simulink model "Switching_07"  (R2022b)
settings: Solver=ode4  StartTime=0.0  StopTime=50  FixedStep=1e-3  MaxStep=1e-3  RelTol=1e-3
undefined symbols (not defined in the file or in its folder): den_filter, der_sat, num_filter, OF_k1_FD, OF_k2_FD, OF_k3_FD, OF_k4_FD, p1, p2, p3, PR_k1, PR_k2, PR_k3, theta_d, tolerance_posture, v_sat, w_sat, x_d, y_d
libraries: simulink x18, dspsigops x3
settings Model: Creator=david  LastModifiedBy=aless

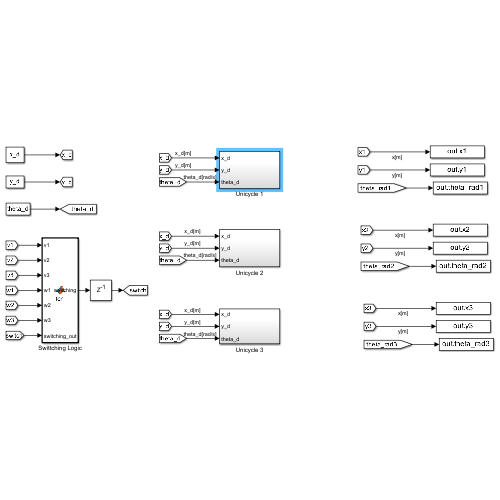
[thumbnail: Simulink's stored preview of the top-level diagram]
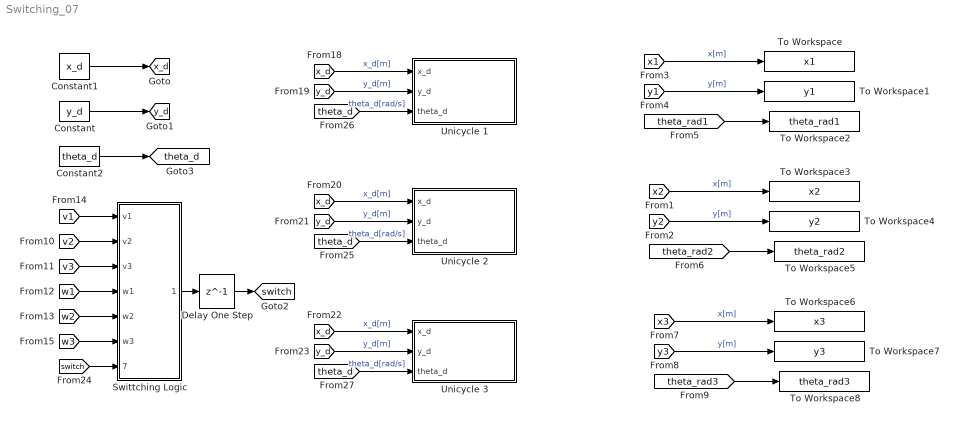
== system Switching_07 ==
  Constant : Constant  Value=y_d
  Constant1 : Constant  Value=x_d
  Constant2 : Constant  Value=theta_d
  Delay One Step : Delay  DelayLength=1
  Swittching Logic : MATLAB Function  TreatAsAtomicUnit=on
  To Workspace : ToWorkspace  VariableName=x1  SaveFormat=Structure With Time  SampleTime=-1
  To Workspace1 : ToWorkspace  VariableName=y1  SaveFormat=Structure With Time  SampleTime=-1
  To Workspace2 : ToWorkspace  VariableName=theta_rad1  SaveFormat=Structure With Time  SampleTime=-1
  To Workspace3 : ToWorkspace  VariableName=x2  SaveFormat=Structure With Time  SampleTime=-1
  To Workspace4 : ToWorkspace  VariableName=y2  SaveFormat=Structure With Time  SampleTime=-1
  To Workspace5 : ToWorkspace  VariableName=theta_rad2  SaveFormat=Structure With Time  SampleTime=-1
  To Workspace6 : ToWorkspace  VariableName=x3  SaveFormat=Structure With Time  SampleTime=-1
  To Workspace7 : ToWorkspace  VariableName=y3  SaveFormat=Structure With Time  SampleTime=-1
  To Workspace8 : ToWorkspace  VariableName=theta_rad3  SaveFormat=Structure With Time  SampleTime=-1
  Unicycle 1 : Subsystem
  Unicycle 2 : Subsystem
  Unicycle 3 : Subsystem
  tag scope: switch=global, theta_d=global, x_d=global, y_d=global
  wires:
  [x1] -> To Workspace/1  "x[m]"
  [y1] -> To Workspace1/1  "y[m]"
  [theta_rad1] -> To Workspace2/1
  [x2] -> To Workspace3/1  "x[m]"
  [y2] -> To Workspace4/1  "y[m]"
  [theta_rad2] -> To Workspace5/1
  [theta_rad3] -> To Workspace8/1
  [y3] -> To Workspace7/1  "y[m]"
  [x3] -> To Workspace6/1  "x[m]"
  [w2] -> Swittching Logic/5(w2)
  [v1] -> Swittching Logic/1(v1)
  [v2] -> Swittching Logic/2(v2)
  Constant2/1 -> [theta_d]
  [w1] -> Swittching Logic/4(w1)
  [v3] -> Swittching Logic/3(v3)
  [x_d] -> Unicycle 1/1(x_d)  "x_d[m]"
  [y_d] -> Unicycle 3/2(y_d)  "y_d[m]"
  [switch] -> Swittching Logic/7(switching_out)
  Swittching Logic/1(switching) -> Delay One Step/1
  [theta_d] -> Unicycle 3/3(theta_d)  "theta_d[rad/s]"
  [x_d] -> Unicycle 2/1(x_d)  "x_d[m]"
  [w3] -> Swittching Logic/6(w3)
  Constant/1 -> [y_d]
  Delay One Step/1 -> [switch]
  [y_d] -> Unicycle 1/2(y_d)  "y_d[m]"
  [theta_d] -> Unicycle 2/3(theta_d)  "theta_d[rad/s]"
  [y_d] -> Unicycle 2/2(y_d)  "y_d[m]"
  [x_d] -> Unicycle 3/1(x_d)  "x_d[m]"
  Constant1/1 -> [x_d]
  [theta_d] -> Unicycle 1/3(theta_d)  "theta_d[rad/s]"

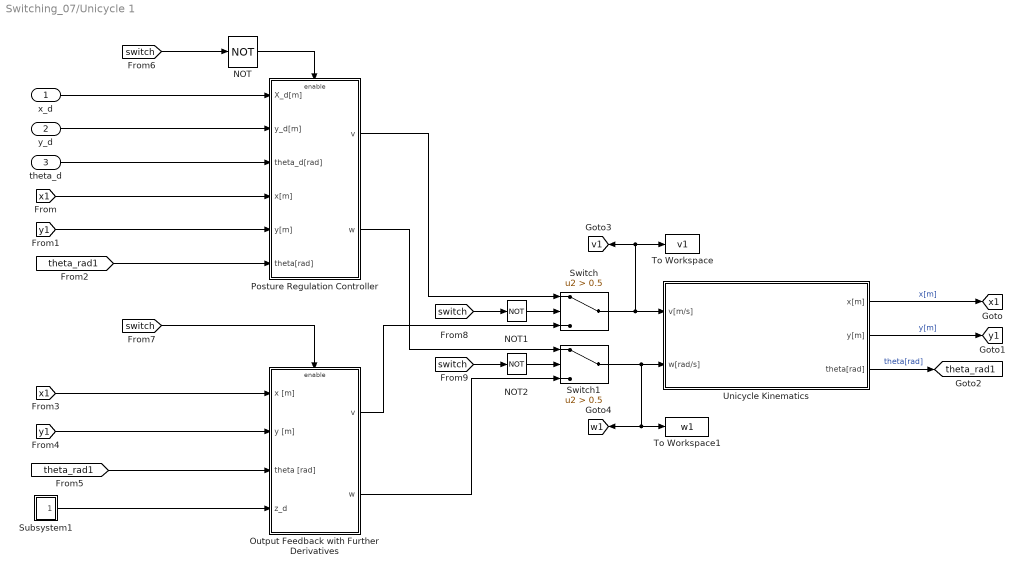
== system Switching_07/Unicycle 1 ==
  x_d : Inport
  y_d : Inport  Port=2
  theta_d : Inport  Port=3
  NOT : Logic  Operator=NOT  IconShape=distinctive  AllPortsSameDT=off  OutDataTypeStr=boolean
  NOT1 : Logic  Operator=NOT  IconShape=distinctive  AllPortsSameDT=off  OutDataTypeStr=boolean
  NOT2 : Logic  Operator=NOT  IconShape=distinctive  AllPortsSameDT=off  OutDataTypeStr=boolean
  Output Feedback with Further Derivatives : Subsystem
  Posture Regulation Controller : Subsystem
  Subsystem1 : Subsystem
  Switch : Switch  Criteria=u2 > Threshold  Threshold=0.5  SaturateOnIntegerOverflow=off  InputSameDT=off
  Switch1 : Switch  Criteria=u2 > Threshold  Threshold=0.5  SaturateOnIntegerOverflow=off  InputSameDT=off
  To Workspace : ToWorkspace  VariableName=v1  SaveFormat=Structure With Time  SampleTime=-1
  To Workspace1 : ToWorkspace  VariableName=w1  SaveFormat=Structure With Time  SampleTime=-1
  Unicycle Kinematics : Subsystem
  tag scope: theta_rad1=global, v1=global, w1=global, x1=global, y1=global
  wires:
  Unicycle Kinematics/3(theta[rad]) -> [theta_rad1]  "theta[rad]"
  Unicycle Kinematics/2(y[m]) -> [y1]  "y[m]"
  Unicycle Kinematics/1(x[m]) -> [x1]  "x[m]"
  [theta_rad1] -> Output Feedback with Further Derivatives/3(theta [rad])
  [x1] -> Output Feedback with Further Derivatives/1(x [m])
  [y1] -> Output Feedback with Further Derivatives/2(y [m])
  [switch] -> Output Feedback with Further Derivatives/Enable
  Posture Regulation Controller/2(w) -> Switch1/1
  Posture Regulation Controller/1(v) -> Switch/1
  Output Feedback with Further Derivatives/2(w) -> Switch1/3
  [switch] -> NOT2/1
  Output Feedback with Further Derivatives/1(v) -> Switch/3
  [switch] -> NOT1/1
  NOT1/1 -> Switch/2
  NOT2/1 -> Switch1/2
  Switch1/1 -> Unicycle Kinematics/2(w[rad/s]), [w1], To Workspace1/1
  Switch/1 -> Unicycle Kinematics/1(v[m/s]), [v1], To Workspace/1
  Subsystem1/1(z_d) -> Output Feedback with Further Derivatives/4(z_d)
  [x1] -> Posture Regulation Controller/4(x[m])
  [switch] -> NOT/1
  x_d/1 -> Posture Regulation Controller/1(X_d[m])
  [theta_rad1] -> Posture Regulation Controller/6(theta[rad])
  [y1] -> Posture Regulation Controller/5(y[m])
  y_d/1 -> Posture Regulation Controller/2(y_d[m])
  NOT/1 -> Posture Regulation Controller/Enable
  theta_d/1 -> Posture Regulation Controller/3(theta_d[rad])

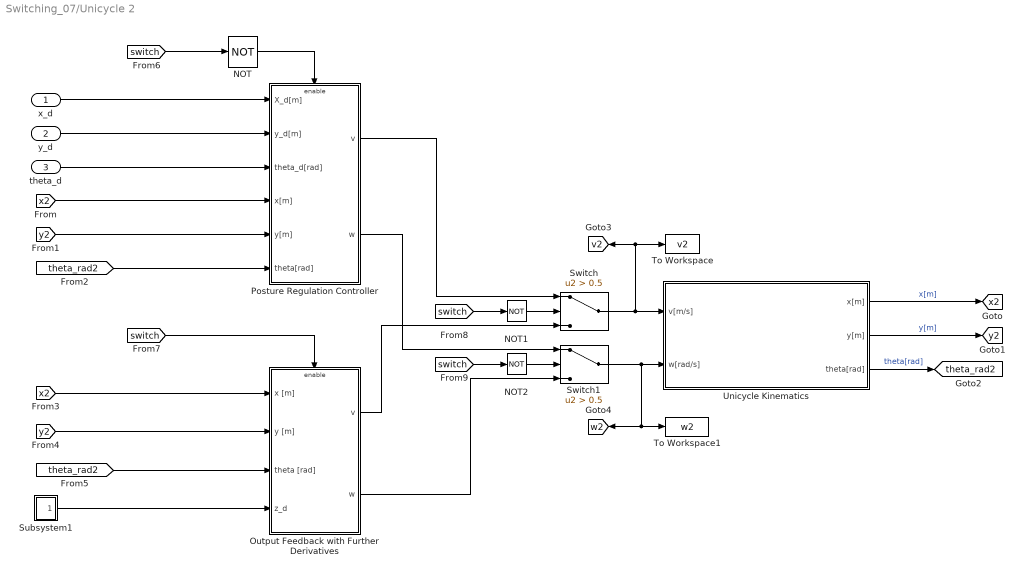
== system Switching_07/Unicycle 2 ==
  x_d : Inport
  y_d : Inport  Port=2
  theta_d : Inport  Port=3
  NOT : Logic  Operator=NOT  IconShape=distinctive  AllPortsSameDT=off  OutDataTypeStr=boolean
  NOT1 : Logic  Operator=NOT  IconShape=distinctive  AllPortsSameDT=off  OutDataTypeStr=boolean
  NOT2 : Logic  Operator=NOT  IconShape=distinctive  AllPortsSameDT=off  OutDataTypeStr=boolean
  Output Feedback with Further Derivatives : Subsystem
  Posture Regulation Controller : Subsystem
  Subsystem1 : Subsystem
  Switch : Switch  Criteria=u2 > Threshold  Threshold=0.5  SaturateOnIntegerOverflow=off  InputSameDT=off
  Switch1 : Switch  Criteria=u2 > Threshold  Threshold=0.5  SaturateOnIntegerOverflow=off  InputSameDT=off
  To Workspace : ToWorkspace  VariableName=v2  SaveFormat=Structure With Time  SampleTime=-1
  To Workspace1 : ToWorkspace  VariableName=w2  SaveFormat=Structure With Time  SampleTime=-1
  Unicycle Kinematics : Subsystem
  tag scope: theta_rad2=global, v2=global, w2=global, x2=global, y2=global
  wires:
  Unicycle Kinematics/3(theta[rad]) -> [theta_rad2]  "theta[rad]"
  Unicycle Kinematics/2(y[m]) -> [y2]  "y[m]"
  Unicycle Kinematics/1(x[m]) -> [x2]  "x[m]"
  [theta_rad2] -> Output Feedback with Further Derivatives/3(theta [rad])
  [x2] -> Output Feedback with Further Derivatives/1(x [m])
  [y2] -> Output Feedback with Further Derivatives/2(y [m])
  [switch] -> Output Feedback with Further Derivatives/Enable
  Posture Regulation Controller/2(w) -> Switch1/1
  Posture Regulation Controller/1(v) -> Switch/1
  Output Feedback with Further Derivatives/2(w) -> Switch1/3
  [switch] -> NOT2/1
  [switch] -> NOT1/1
  NOT1/1 -> Switch/2
  NOT2/1 -> Switch1/2
  Output Feedback with Further Derivatives/1(v) -> Switch/3
  Switch1/1 -> Unicycle Kinematics/2(w[rad/s]), To Workspace1/1, [w2]
  Switch/1 -> Unicycle Kinematics/1(v[m/s]), [v2], To Workspace/1
  Subsystem1/1(z_d) -> Output Feedback with Further Derivatives/4(z_d)
  theta_d/1 -> Posture Regulation Controller/3(theta_d[rad])
  x_d/1 -> Posture Regulation Controller/1(X_d[m])
  [switch] -> NOT/1
  [x2] -> Posture Regulation Controller/4(x[m])
  [y2] -> Posture Regulation Controller/5(y[m])
  NOT/1 -> Posture Regulation Controller/Enable
  y_d/1 -> Posture Regulation Controller/2(y_d[m])
  [theta_rad2] -> Posture Regulation Controller/6(theta[rad])

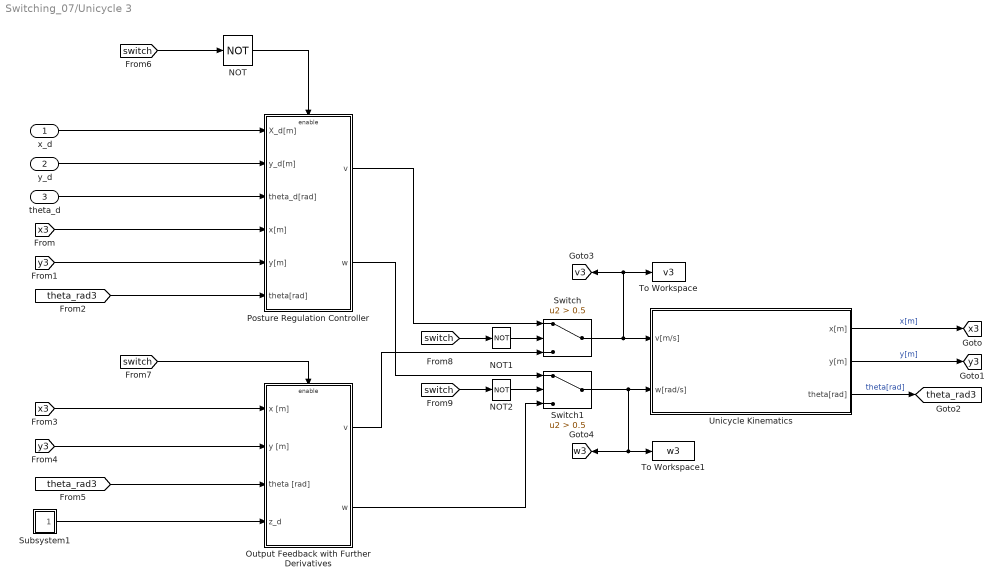
== system Switching_07/Unicycle 3 ==
  x_d : Inport
  y_d : Inport  Port=2
  theta_d : Inport  Port=3
  NOT : Logic  Operator=NOT  IconShape=distinctive  AllPortsSameDT=off  OutDataTypeStr=boolean
  NOT1 : Logic  Operator=NOT  IconShape=distinctive  AllPortsSameDT=off  OutDataTypeStr=boolean
  NOT2 : Logic  Operator=NOT  IconShape=distinctive  AllPortsSameDT=off  OutDataTypeStr=boolean
  Output Feedback with Further Derivatives : Subsystem
  Posture Regulation Controller : Subsystem
  Subsystem1 : Subsystem
  Switch : Switch  Criteria=u2 > Threshold  Threshold=0.5  SaturateOnIntegerOverflow=off  InputSameDT=off
  Switch1 : Switch  Criteria=u2 > Threshold  Threshold=0.5  SaturateOnIntegerOverflow=off  InputSameDT=off
  To Workspace : ToWorkspace  VariableName=v3  SaveFormat=Structure With Time  SampleTime=-1
  To Workspace1 : ToWorkspace  VariableName=w3  SaveFormat=Structure With Time  SampleTime=-1
  Unicycle Kinematics : Subsystem
  tag scope: theta_rad3=global, v3=global, w3=global, x3=global, y3=global
  wires:
  Unicycle Kinematics/3(theta[rad]) -> [theta_rad3]  "theta[rad]"
  Unicycle Kinematics/2(y[m]) -> [y3]  "y[m]"
  Unicycle Kinematics/1(x[m]) -> [x3]  "x[m]"
  [switch] -> Output Feedback with Further Derivatives/Enable
  Posture Regulation Controller/1(v) -> Switch/1
  Output Feedback with Further Derivatives/1(v) -> Switch/3
  Posture Regulation Controller/2(w) -> Switch1/1
  Output Feedback with Further Derivatives/2(w) -> Switch1/3
  NOT1/1 -> Switch/2
  NOT2/1 -> Switch1/2
  Switch1/1 -> Unicycle Kinematics/2(w[rad/s]), To Workspace1/1, [w3]
  Switch/1 -> Unicycle Kinematics/1(v[m/s]), To Workspace/1, [v3]
  [x3] -> Output Feedback with Further Derivatives/1(x [m])
  [y3] -> Output Feedback with Further Derivatives/2(y [m])
  [theta_rad3] -> Output Feedback with Further Derivatives/3(theta [rad])
  Subsystem1/1(z_d) -> Output Feedback with Further Derivatives/4(z_d)
  [switch] -> NOT2/1
  [switch] -> NOT1/1
  y_d/1 -> Posture Regulation Controller/2(y_d[m])
  [y3] -> Posture Regulation Controller/5(y[m])
  [x3] -> Posture Regulation Controller/4(x[m])
  x_d/1 -> Posture Regulation Controller/1(X_d[m])
  theta_d/1 -> Posture Regulation Controller/3(theta_d[rad])
  [switch] -> NOT/1
  NOT/1 -> Posture Regulation Controller/Enable
  [theta_rad3] -> Posture Regulation Controller/6(theta[rad])

== system Switching_07/Unicycle 1/Output Feedback with Further Derivatives ==
  x [m] : Inport
  y [m] : Inport  Port=2
  theta [rad] : Inport  Port=3
  z_d : Inport  Port=4
  Enable : EnablePort
  Inverse transformation : Subsystem
  Subsystem2 : Subsystem
  v : Outport
  w : Outport  Port=2
  wires:
  Subsystem2/1(v) -> v/1
  Subsystem2/2(w) -> w/1
  z_d/1 -> Subsystem2/1(z_d)
  x [m]/1 -> Inverse transformation/1(x)
  y [m]/1 -> Inverse transformation/2(y)
  Inverse transformation/1(z) -> Subsystem2/2(z)
  theta [rad]/1 -> Subsystem2/3(theta_rad)

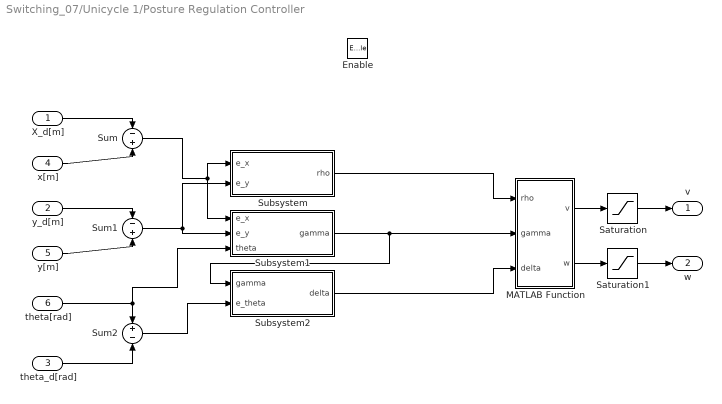
== system Switching_07/Unicycle 1/Posture Regulation Controller ==
  X_d[m] : Inport
  y_d[m] : Inport  Port=2
  theta_d[rad] : Inport  Port=3
  x[m] : Inport  Port=4
  y[m] : Inport  Port=5
  theta[rad] : Inport  Port=6
  Enable : EnablePort
  MATLAB Function : MATLAB Function  TreatAsAtomicUnit=on
  Saturation : Saturate  UpperLimit=v_sat  LowerLimit=-v_sat
  Saturation1 : Saturate  UpperLimit=w_sat  LowerLimit=-w_sat
  Subsystem : Subsystem
  Subsystem1 : Subsystem
  Subsystem2 : Subsystem
  Sum : Sum  Inputs=-+
  Sum1 : Sum  Inputs=-+
  Sum2 : Sum  Inputs=+-
  v : Outport
  w : Outport  Port=2
  wires:
  X_d[m]/1 -> Sum/1
  x[m]/1 -> Sum/2
  y_d[m]/1 -> Sum1/1
  y[m]/1 -> Sum1/2
  Sum1/1 -> Subsystem1/2(e_y), Subsystem/2(e_y)
  Sum2/1 -> Subsystem2/2(e_theta)
  Subsystem1/1(gamma) -> MATLAB Function/2(gamma), Subsystem2/1(gamma)
  Subsystem2/1(delta) -> MATLAB Function/3(delta)
  Subsystem/1(rho) -> MATLAB Function/1(rho)
  Sum/1 -> Subsystem1/1(e_x), Subsystem/1(e_x)
  MATLAB Function/1(v) -> Saturation/1
  MATLAB Function/2(w) -> Saturation1/1
  theta[rad]/1 -> Sum2/1, Subsystem1/3(theta)
  theta_d[rad]/1 -> Sum2/2
  Saturation1/1 -> w/1
  Saturation/1 -> v/1

== system Switching_07/Unicycle 1/Subsystem1 ==
  Mux : Mux
  Repeating Sequence : simulink/Sources/Repeating Sequence  rep_seq_t=time  rep_seq_y=y_d1
  Repeating Sequence1 : simulink/Sources/Repeating Sequence  rep_seq_t=time  rep_seq_y=x_d1
  To Workspace2 : ToWorkspace  VariableName=y_d1  SaveFormat=Structure With Time  SampleTime=-1
  To Workspace3 : ToWorkspace  VariableName=x_d1  SaveFormat=Structure With Time  SampleTime=-1
  x_dot1 : simulink/Sources/Repeating Sequence  rep_seq_t=time  rep_seq_y=x_dot1
  y_dot1 : simulink/Sources/Repeating Sequence  rep_seq_t=time  rep_seq_y=y_dot1
  z_d : Outport
  wires:
  Repeating Sequence1/1 -> To Workspace3/1, Mux/1
  Repeating Sequence/1 -> To Workspace2/1, Mux/2
  Mux/1 -> z_d/1
  x_dot1/1 -> Mux/3
  y_dot1/1 -> Mux/4

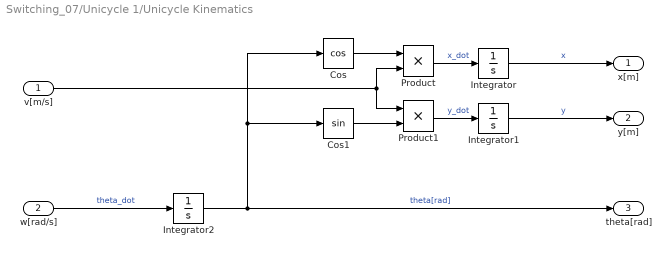
== system Switching_07/Unicycle 1/Unicycle Kinematics ==
  v[m/s] : Inport
  w[rad/s] : Inport  Port=2
  Cos : Trigonometry  Operator=cos
  Cos1 : Trigonometry
  Integrator : Integrator  InitialCondition=p1(1)
  Integrator1 : Integrator  InitialCondition=p1(2)
  Integrator2 : Integrator  InitialCondition=p1(3)
  Product : Product
  Product1 : Product
  x[m] : Outport
  y[m] : Outport  Port=2
  theta[rad] : Outport  Port=3
  wires:
  Integrator/1 -> x[m]/1  "x"
  Integrator1/1 -> y[m]/1  "y"
  w[rad/s]/1 -> Integrator2/1  "theta_dot"
  Integrator2/1 -> Cos/1, Cos1/1, theta[rad]/1  "theta[rad]"
  Product/1 -> Integrator/1  "x_dot"
  Cos1/1 -> Product1/2
  Cos/1 -> Product/1
  v[m/s]/1 -> Product1/1, Product/2
  Product1/1 -> Integrator1/1  "y_dot"

== system Switching_07/Unicycle 2/Output Feedback with Further Derivatives ==
  x [m] : Inport
  y [m] : Inport  Port=2
  theta [rad] : Inport  Port=3
  z_d : Inport  Port=4
  Enable : EnablePort
  Inverse transformation : Subsystem
  Subsystem2 : Subsystem
  v : Outport
  w : Outport  Port=2
  wires:
  Subsystem2/1(v) -> v/1
  Subsystem2/2(w) -> w/1
  z_d/1 -> Subsystem2/1(z_d)
  x [m]/1 -> Inverse transformation/1(x)
  y [m]/1 -> Inverse transformation/2(y)
  Inverse transformation/1(z) -> Subsystem2/2(z)
  theta [rad]/1 -> Subsystem2/3(theta_rad)

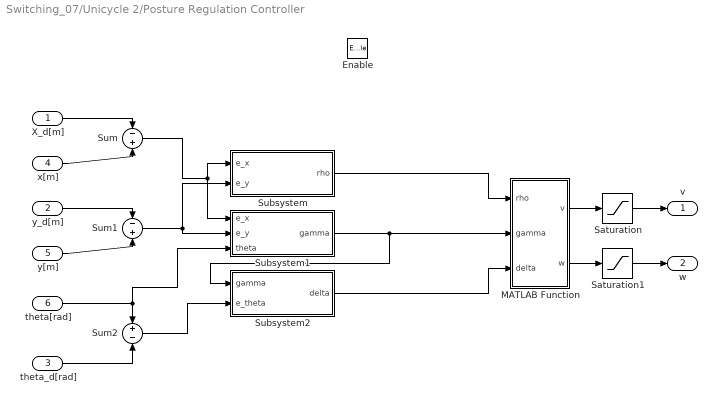
== system Switching_07/Unicycle 2/Posture Regulation Controller ==
  X_d[m] : Inport
  y_d[m] : Inport  Port=2
  theta_d[rad] : Inport  Port=3
  x[m] : Inport  Port=4
  y[m] : Inport  Port=5
  theta[rad] : Inport  Port=6
  Enable : EnablePort
  MATLAB Function : MATLAB Function  TreatAsAtomicUnit=on
  Saturation : Saturate  UpperLimit=v_sat  LowerLimit=-v_sat
  Saturation1 : Saturate  UpperLimit=w_sat  LowerLimit=-w_sat
  Subsystem : Subsystem
  Subsystem1 : Subsystem
  Subsystem2 : Subsystem
  Sum : Sum  Inputs=-+
  Sum1 : Sum  Inputs=-+
  Sum2 : Sum  Inputs=+-
  v : Outport
  w : Outport  Port=2
  wires:
  X_d[m]/1 -> Sum/1
  x[m]/1 -> Sum/2
  y_d[m]/1 -> Sum1/1
  y[m]/1 -> Sum1/2
  Sum1/1 -> Subsystem1/2(e_y), Subsystem/2(e_y)
  Sum2/1 -> Subsystem2/2(e_theta)
  Subsystem1/1(gamma) -> MATLAB Function/2(gamma), Subsystem2/1(gamma)
  Subsystem2/1(delta) -> MATLAB Function/3(delta)
  Subsystem/1(rho) -> MATLAB Function/1(rho)
  Sum/1 -> Subsystem1/1(e_x), Subsystem/1(e_x)
  MATLAB Function/1(v) -> Saturation/1
  MATLAB Function/2(w) -> Saturation1/1
  theta[rad]/1 -> Sum2/1, Subsystem1/3(theta)
  theta_d[rad]/1 -> Sum2/2
  Saturation/1 -> v/1
  Saturation1/1 -> w/1

== system Switching_07/Unicycle 2/Subsystem1 ==
  Mux : Mux
  Repeating Sequence : simulink/Sources/Repeating Sequence  rep_seq_t=time  rep_seq_y=y_d2
  Repeating Sequence1 : simulink/Sources/Repeating Sequence  rep_seq_t=time  rep_seq_y=x_d2
  To Workspace2 : ToWorkspace  VariableName=y_d2  SaveFormat=Structure With Time  SampleTime=-1
  To Workspace3 : ToWorkspace  VariableName=x_d2  SaveFormat=Structure With Time  SampleTime=-1
  x_dot1 : simulink/Sources/Repeating Sequence  rep_seq_t=time  rep_seq_y=x_dot2
  y_dot1 : simulink/Sources/Repeating Sequence  rep_seq_t=time  rep_seq_y=y_dot2
  z_d : Outport
  wires:
  Repeating Sequence1/1 -> To Workspace3/1, Mux/1
  Repeating Sequence/1 -> To Workspace2/1, Mux/2
  Mux/1 -> z_d/1
  x_dot1/1 -> Mux/3
  y_dot1/1 -> Mux/4

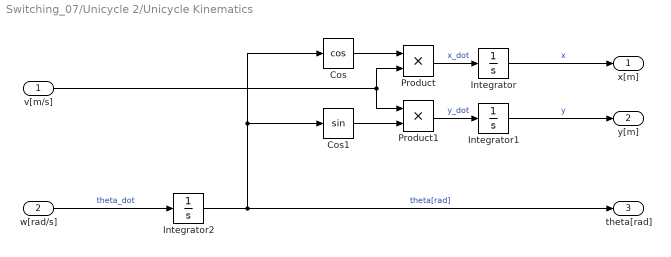
== system Switching_07/Unicycle 2/Unicycle Kinematics ==
  v[m/s] : Inport
  w[rad/s] : Inport  Port=2
  Cos : Trigonometry  Operator=cos
  Cos1 : Trigonometry
  Integrator : Integrator  InitialCondition=p2(1)
  Integrator1 : Integrator  InitialCondition=p2(2)
  Integrator2 : Integrator  InitialCondition=p2(3)
  Product : Product
  Product1 : Product
  x[m] : Outport
  y[m] : Outport  Port=2
  theta[rad] : Outport  Port=3
  wires:
  Integrator/1 -> x[m]/1  "x"
  Integrator1/1 -> y[m]/1  "y"
  w[rad/s]/1 -> Integrator2/1  "theta_dot"
  Integrator2/1 -> Cos/1, Cos1/1, theta[rad]/1  "theta[rad]"
  Product/1 -> Integrator/1  "x_dot"
  Cos1/1 -> Product1/2
  Cos/1 -> Product/1
  v[m/s]/1 -> Product1/1, Product/2
  Product1/1 -> Integrator1/1  "y_dot"

== system Switching_07/Unicycle 3/Output Feedback with Further Derivatives ==
  x [m] : Inport
  y [m] : Inport  Port=2
  theta [rad] : Inport  Port=3
  z_d : Inport  Port=4
  Enable : EnablePort
  Inverse transformation : Subsystem
  Subsystem2 : Subsystem
  v : Outport
  w : Outport  Port=2
  wires:
  Subsystem2/1(v) -> v/1
  Subsystem2/2(w) -> w/1
  z_d/1 -> Subsystem2/1(z_d)
  x [m]/1 -> Inverse transformation/1(x)
  y [m]/1 -> Inverse transformation/2(y)
  Inverse transformation/1(z) -> Subsystem2/2(z)
  theta [rad]/1 -> Subsystem2/3(theta_rad)

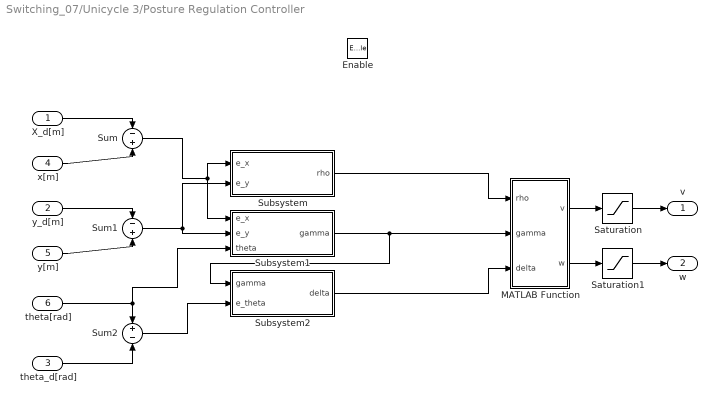
== system Switching_07/Unicycle 3/Posture Regulation Controller ==
  X_d[m] : Inport
  y_d[m] : Inport  Port=2
  theta_d[rad] : Inport  Port=3
  x[m] : Inport  Port=4
  y[m] : Inport  Port=5
  theta[rad] : Inport  Port=6
  Enable : EnablePort
  MATLAB Function : MATLAB Function  TreatAsAtomicUnit=on
  Saturation : Saturate  UpperLimit=v_sat  LowerLimit=-v_sat
  Saturation1 : Saturate  UpperLimit=w_sat  LowerLimit=-w_sat
  Subsystem : Subsystem
  Subsystem1 : Subsystem
  Subsystem2 : Subsystem
  Sum : Sum  Inputs=-+
  Sum1 : Sum  Inputs=-+
  Sum2 : Sum  Inputs=+-
  v : Outport
  w : Outport  Port=2
  wires:
  X_d[m]/1 -> Sum/1
  x[m]/1 -> Sum/2
  y_d[m]/1 -> Sum1/1
  y[m]/1 -> Sum1/2
  Sum1/1 -> Subsystem1/2(e_y), Subsystem/2(e_y)
  Sum2/1 -> Subsystem2/2(e_theta)
  Subsystem1/1(gamma) -> MATLAB Function/2(gamma), Subsystem2/1(gamma)
  Subsystem2/1(delta) -> MATLAB Function/3(delta)
  Subsystem/1(rho) -> MATLAB Function/1(rho)
  Sum/1 -> Subsystem1/1(e_x), Subsystem/1(e_x)
  MATLAB Function/1(v) -> Saturation/1
  MATLAB Function/2(w) -> Saturation1/1
  theta[rad]/1 -> Sum2/1, Subsystem1/3(theta)
  theta_d[rad]/1 -> Sum2/2
  Saturation1/1 -> w/1
  Saturation/1 -> v/1

== system Switching_07/Unicycle 3/Subsystem1 ==
  Mux : Mux
  Repeating Sequence : simulink/Sources/Repeating Sequence  rep_seq_t=time  rep_seq_y=y_d3
  Repeating Sequence1 : simulink/Sources/Repeating Sequence  rep_seq_t=time  rep_seq_y=x_d3
  To Workspace2 : ToWorkspace  VariableName=y_d3  SaveFormat=Structure With Time  SampleTime=-1
  To Workspace3 : ToWorkspace  VariableName=x_d3  SaveFormat=Structure With Time  SampleTime=-1
  x_dot1 : simulink/Sources/Repeating Sequence  rep_seq_t=time  rep_seq_y=x_dot3
  y_dot1 : simulink/Sources/Repeating Sequence  rep_seq_t=time  rep_seq_y=y_dot3
  z_d : Outport
  wires:
  Repeating Sequence1/1 -> To Workspace3/1, Mux/1
  Repeating Sequence/1 -> To Workspace2/1, Mux/2
  Mux/1 -> z_d/1
  x_dot1/1 -> Mux/3
  y_dot1/1 -> Mux/4

== system Switching_07/Unicycle 3/Unicycle Kinematics ==
  v[m/s] : Inport
  w[rad/s] : Inport  Port=2
  Cos : Trigonometry  Operator=cos
  Cos1 : Trigonometry
  Integrator : Integrator  InitialCondition=p3(1)
  Integrator1 : Integrator  InitialCondition=p3(2)
  Integrator2 : Integrator  InitialCondition=p3(3)
  Product : Product
  Product1 : Product
  x[m] : Outport
  y[m] : Outport  Port=2
  theta[rad] : Outport  Port=3
  wires:
  Integrator/1 -> x[m]/1  "x"
  Integrator1/1 -> y[m]/1  "y"
  w[rad/s]/1 -> Integrator2/1  "theta_dot"
  Integrator2/1 -> Cos/1, Cos1/1, theta[rad]/1  "theta[rad]"
  Product/1 -> Integrator/1  "x_dot"
  Cos1/1 -> Product1/2
  Cos/1 -> Product/1
  v[m/s]/1 -> Product1/1, Product/2
  Product1/1 -> Integrator1/1  "y_dot"

== system Switching_07/Unicycle 1/Output Feedback with Further Derivatives/Inverse transformation ==
  x : Inport
  y : Inport  Port=2
  Mux : Mux
  Saturation1 : Saturate  UpperLimit=der_sat  LowerLimit=-der_sat
  Saturation2 : Saturate  UpperLimit=der_sat  LowerLimit=-der_sat
  Transfer Fcn : TransferFcn  Numerator=num_filter  Denominator=den_filter
  Transfer Fcn1 : TransferFcn  Numerator=num_filter  Denominator=den_filter
  z : Outport
  wires:
  Mux/1 -> z/1
  x/1 -> Transfer Fcn/1, Mux/1
  y/1 -> Transfer Fcn1/1, Mux/2
  Transfer Fcn/1 -> Saturation1/1
  Transfer Fcn1/1 -> Saturation2/1
  Saturation1/1 -> Mux/3
  Saturation2/1 -> Mux/4

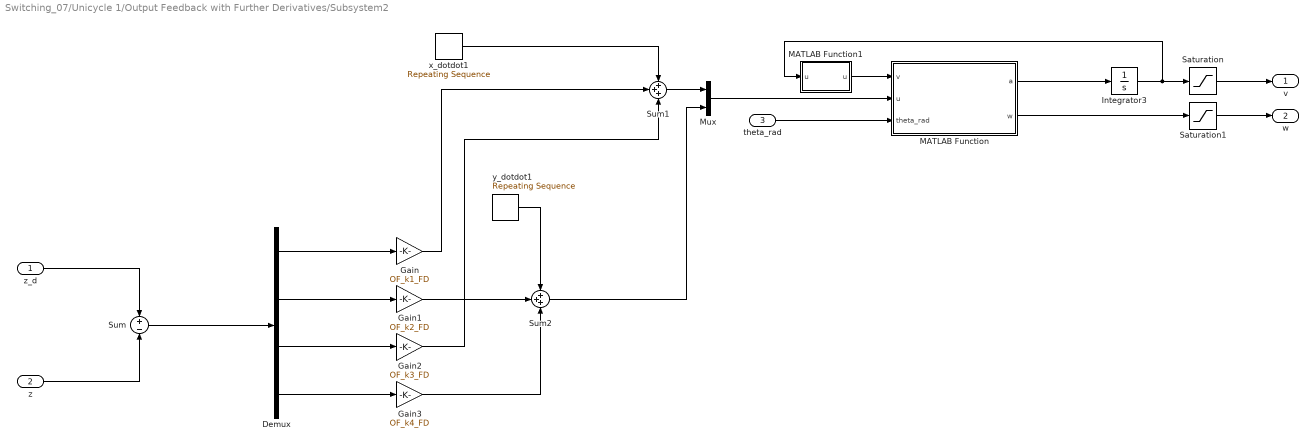
== system Switching_07/Unicycle 1/Output Feedback with Further Derivatives/Subsystem2 ==
  z_d : Inport
  z : Inport  Port=2
  theta_rad : Inport  Port=3
  Demux : Demux
  Gain : Gain  Gain=OF_k1_FD
  Gain1 : Gain  Gain=OF_k2_FD
  Gain2 : Gain  Gain=OF_k3_FD
  Gain3 : Gain  Gain=OF_k4_FD
  Integrator3 : Integrator  InitialCondition=1e-4
  MATLAB Function : MATLAB Function  TreatAsAtomicUnit=on
  MATLAB Function1 : MATLAB Function  TreatAsAtomicUnit=on
  Mux : Mux  Inputs=2
  Saturation : Saturate  UpperLimit=v_sat  LowerLimit=-v_sat
  Saturation1 : Saturate  UpperLimit=w_sat  LowerLimit=-w_sat
  Sum : Sum  Inputs=+-
  Sum1 : Sum  Inputs=+++
  Sum2 : Sum  Inputs=+++
  x_dotdot1 : simulink/Sources/Repeating Sequence  rep_seq_t=time  rep_seq_y=x_dotdot1
  y_dotdot1 : simulink/Sources/Repeating Sequence  rep_seq_t=time  rep_seq_y=y_dotdot1
  v : Outport
  w : Outport  Port=2
  wires:
  z_d/1 -> Sum/1
  z/1 -> Sum/2
  Sum/1 -> Demux/1
  Demux/1 -> Gain/1
  Demux/2 -> Gain1/1
  Demux/3 -> Gain2/1
  Demux/4 -> Gain3/1
  x_dotdot1/1 -> Sum1/1
  Sum1/1 -> Mux/1
  Mux/1 -> MATLAB Function/2(u)
  Gain/1 -> Sum1/2
  y_dotdot1/1 -> Sum2/1
  Sum2/1 -> Mux/2
  theta_rad/1 -> MATLAB Function/3(theta_rad)
  MATLAB Function/1(a) -> Integrator3/1
  MATLAB Function/2(w) -> Saturation1/1
  MATLAB Function1/1(u) -> MATLAB Function/1(v)
  Gain2/1 -> Sum1/3
  Gain1/1 -> Sum2/2
  Gain3/1 -> Sum2/3
  Integrator3/1 -> Saturation/1, MATLAB Function1/1("u ")
  Saturation/1 -> v/1
  Saturation1/1 -> w/1

== system Switching_07/Unicycle 1/Posture Regulation Controller/Subsystem ==
  e_x : Inport
  e_y : Inport  Port=2
  Sqrt : Sqrt
  Square : Math  Operator=square
  Square1 : Math  Operator=square
  Sum : Sum
  rho : Outport
  wires:
  Sqrt/1 -> rho/1
  e_x/1 -> Square/1
  e_y/1 -> Square1/1
  Sum/1 -> Sqrt/1
  Square/1 -> Sum/1
  Square1/1 -> Sum/2

== system Switching_07/Unicycle 1/Posture Regulation Controller/Subsystem1 ==
  e_x : Inport
  e_y : Inport  Port=2
  theta : Inport  Port=3
  Atan2 : Trigonometry  Operator=atan2
  Constant : Constant  Value=pi
  Sum : Sum  Inputs=+-+
  Unwrap : dspsigops/Unwrap  tol=pi  InputProcessing=Columns as channels (frame based)  running=off
  gamma : Outport
  wires:
  e_x/1 -> Atan2/2
  e_y/1 -> Atan2/1
  theta/1 -> Sum/2
  Sum/1 -> gamma/1
  Atan2/1 -> Unwrap/1
  Constant/1 -> Sum/3
  Unwrap/1 -> Sum/1

== system Switching_07/Unicycle 1/Posture Regulation Controller/Subsystem2 ==
  gamma : Inport
  e_theta : Inport  Port=2
  Sum : Sum
  delta : Outport
  wires:
  e_theta/1 -> Sum/2
  Sum/1 -> delta/1
  gamma/1 -> Sum/1

== system Switching_07/Unicycle 2/Output Feedback with Further Derivatives/Inverse transformation ==
  x : Inport
  y : Inport  Port=2
  Mux : Mux
  Saturation1 : Saturate  UpperLimit=der_sat  LowerLimit=-der_sat
  Saturation2 : Saturate  UpperLimit=der_sat  LowerLimit=-der_sat
  Transfer Fcn : TransferFcn  Numerator=num_filter  Denominator=den_filter
  Transfer Fcn1 : TransferFcn  Numerator=num_filter  Denominator=den_filter
  z : Outport
  wires:
  Mux/1 -> z/1
  x/1 -> Transfer Fcn/1, Mux/1
  y/1 -> Transfer Fcn1/1, Mux/2
  Transfer Fcn/1 -> Saturation1/1
  Transfer Fcn1/1 -> Saturation2/1
  Saturation2/1 -> Mux/4
  Saturation1/1 -> Mux/3

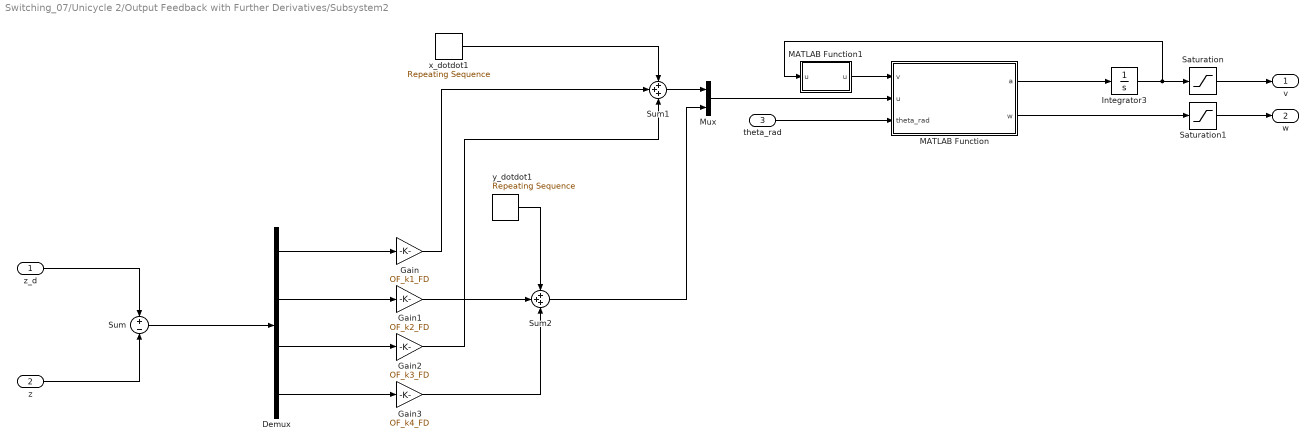
== system Switching_07/Unicycle 2/Output Feedback with Further Derivatives/Subsystem2 ==
  z_d : Inport
  z : Inport  Port=2
  theta_rad : Inport  Port=3
  Demux : Demux
  Gain : Gain  Gain=OF_k1_FD
  Gain1 : Gain  Gain=OF_k2_FD
  Gain2 : Gain  Gain=OF_k3_FD
  Gain3 : Gain  Gain=OF_k4_FD
  Integrator3 : Integrator  InitialCondition=1e-4
  MATLAB Function : MATLAB Function  TreatAsAtomicUnit=on
  MATLAB Function1 : MATLAB Function  TreatAsAtomicUnit=on
  Mux : Mux  Inputs=2
  Saturation : Saturate  UpperLimit=v_sat  LowerLimit=-v_sat
  Saturation1 : Saturate  UpperLimit=w_sat  LowerLimit=-w_sat
  Sum : Sum  Inputs=+-
  Sum1 : Sum  Inputs=+++
  Sum2 : Sum  Inputs=+++
  x_dotdot1 : simulink/Sources/Repeating Sequence  rep_seq_t=time  rep_seq_y=x_dotdot2
  y_dotdot1 : simulink/Sources/Repeating Sequence  rep_seq_t=time  rep_seq_y=y_dotdot2
  v : Outport
  w : Outport  Port=2
  wires:
  z_d/1 -> Sum/1
  z/1 -> Sum/2
  Sum/1 -> Demux/1
  Demux/1 -> Gain/1
  Demux/2 -> Gain1/1
  Demux/3 -> Gain2/1
  Demux/4 -> Gain3/1
  x_dotdot1/1 -> Sum1/1
  Sum1/1 -> Mux/1
  Mux/1 -> MATLAB Function/2(u)
  Gain/1 -> Sum1/2
  y_dotdot1/1 -> Sum2/1
  Sum2/1 -> Mux/2
  theta_rad/1 -> MATLAB Function/3(theta_rad)
  MATLAB Function/1(a) -> Integrator3/1
  MATLAB Function/2(w) -> Saturation1/1
  MATLAB Function1/1(u) -> MATLAB Function/1(v)
  Gain2/1 -> Sum1/3
  Gain1/1 -> Sum2/2
  Gain3/1 -> Sum2/3
  Integrator3/1 -> Saturation/1, MATLAB Function1/1("u ")
  Saturation/1 -> v/1
  Saturation1/1 -> w/1

== system Switching_07/Unicycle 2/Posture Regulation Controller/Subsystem ==
  e_x : Inport
  e_y : Inport  Port=2
  Sqrt : Sqrt
  Square : Math  Operator=square
  Square1 : Math  Operator=square
  Sum : Sum
  rho : Outport
  wires:
  Sqrt/1 -> rho/1
  e_x/1 -> Square/1
  e_y/1 -> Square1/1
  Sum/1 -> Sqrt/1
  Square/1 -> Sum/1
  Square1/1 -> Sum/2

== system Switching_07/Unicycle 2/Posture Regulation Controller/Subsystem1 ==
  e_x : Inport
  e_y : Inport  Port=2
  theta : Inport  Port=3
  Atan2 : Trigonometry  Operator=atan2
  Constant : Constant  Value=pi
  Sum : Sum  Inputs=+-+
  Unwrap : dspsigops/Unwrap  tol=pi  InputProcessing=Columns as channels (frame based)  running=off
  gamma : Outport
  wires:
  e_x/1 -> Atan2/2
  e_y/1 -> Atan2/1
  theta/1 -> Sum/2
  Sum/1 -> gamma/1
  Atan2/1 -> Unwrap/1
  Constant/1 -> Sum/3
  Unwrap/1 -> Sum/1

== system Switching_07/Unicycle 2/Posture Regulation Controller/Subsystem2 ==
  gamma : Inport
  e_theta : Inport  Port=2
  Sum : Sum
  delta : Outport
  wires:
  e_theta/1 -> Sum/2
  Sum/1 -> delta/1
  gamma/1 -> Sum/1

== system Switching_07/Unicycle 3/Output Feedback with Further Derivatives/Inverse transformation ==
  x : Inport
  y : Inport  Port=2
  Mux : Mux
  Saturation1 : Saturate  UpperLimit=der_sat  LowerLimit=-der_sat
  Saturation2 : Saturate  UpperLimit=der_sat  LowerLimit=-der_sat
  Transfer Fcn : TransferFcn  Numerator=num_filter  Denominator=den_filter
  Transfer Fcn1 : TransferFcn  Numerator=num_filter  Denominator=den_filter
  z : Outport
  wires:
  Mux/1 -> z/1
  x/1 -> Transfer Fcn/1, Mux/1
  y/1 -> Transfer Fcn1/1, Mux/2
  Transfer Fcn/1 -> Saturation1/1
  Transfer Fcn1/1 -> Saturation2/1
  Saturation2/1 -> Mux/4
  Saturation1/1 -> Mux/3

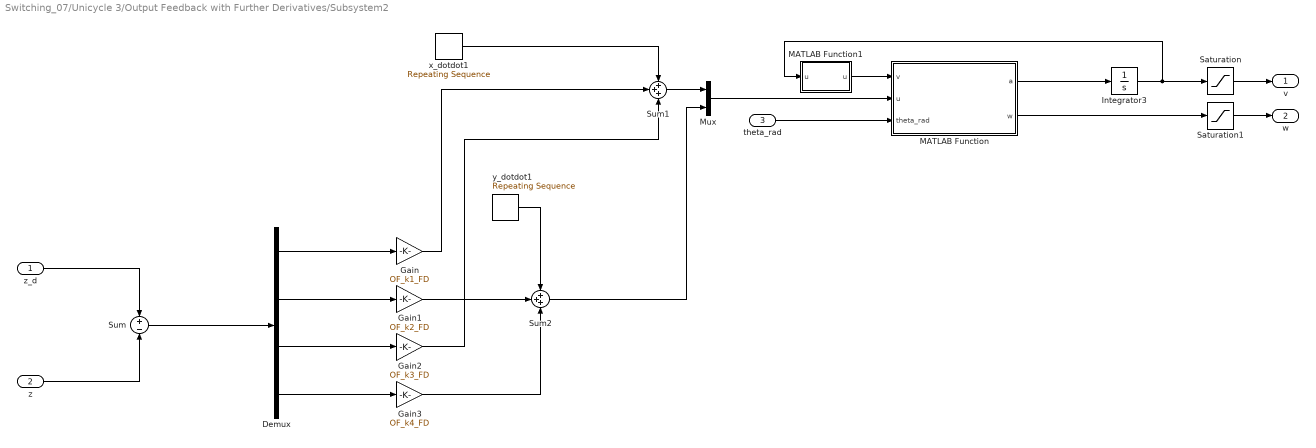
== system Switching_07/Unicycle 3/Output Feedback with Further Derivatives/Subsystem2 ==
  z_d : Inport
  z : Inport  Port=2
  theta_rad : Inport  Port=3
  Demux : Demux
  Gain : Gain  Gain=OF_k1_FD
  Gain1 : Gain  Gain=OF_k2_FD
  Gain2 : Gain  Gain=OF_k3_FD
  Gain3 : Gain  Gain=OF_k4_FD
  Integrator3 : Integrator  InitialCondition=1e-4
  MATLAB Function : MATLAB Function  TreatAsAtomicUnit=on
  MATLAB Function1 : MATLAB Function  TreatAsAtomicUnit=on
  Mux : Mux  Inputs=2
  Saturation : Saturate  UpperLimit=v_sat  LowerLimit=-v_sat
  Saturation1 : Saturate  UpperLimit=w_sat  LowerLimit=-w_sat
  Sum : Sum  Inputs=+-
  Sum1 : Sum  Inputs=+++
  Sum2 : Sum  Inputs=+++
  x_dotdot1 : simulink/Sources/Repeating Sequence  rep_seq_t=time  rep_seq_y=x_dotdot3
  y_dotdot1 : simulink/Sources/Repeating Sequence  rep_seq_t=time  rep_seq_y=y_dotdot3
  v : Outport
  w : Outport  Port=2
  wires:
  z_d/1 -> Sum/1
  z/1 -> Sum/2
  Sum/1 -> Demux/1
  Demux/1 -> Gain/1
  Demux/2 -> Gain1/1
  Demux/3 -> Gain2/1
  Demux/4 -> Gain3/1
  x_dotdot1/1 -> Sum1/1
  Sum1/1 -> Mux/1
  Mux/1 -> MATLAB Function/2(u)
  Gain/1 -> Sum1/2
  y_dotdot1/1 -> Sum2/1
  Sum2/1 -> Mux/2
  theta_rad/1 -> MATLAB Function/3(theta_rad)
  MATLAB Function/1(a) -> Integrator3/1
  MATLAB Function/2(w) -> Saturation1/1
  MATLAB Function1/1(u) -> MATLAB Function/1(v)
  Gain2/1 -> Sum1/3
  Gain1/1 -> Sum2/2
  Gain3/1 -> Sum2/3
  Integrator3/1 -> Saturation/1, MATLAB Function1/1("u ")
  Saturation/1 -> v/1
  Saturation1/1 -> w/1

== system Switching_07/Unicycle 3/Posture Regulation Controller/Subsystem ==
  e_x : Inport
  e_y : Inport  Port=2
  Sqrt : Sqrt
  Square : Math  Operator=square
  Square1 : Math  Operator=square
  Sum : Sum
  rho : Outport
  wires:
  Sqrt/1 -> rho/1
  e_x/1 -> Square/1
  e_y/1 -> Square1/1
  Sum/1 -> Sqrt/1
  Square/1 -> Sum/1
  Square1/1 -> Sum/2

== system Switching_07/Unicycle 3/Posture Regulation Controller/Subsystem1 ==
  e_x : Inport
  e_y : Inport  Port=2
  theta : Inport  Port=3
  Atan2 : Trigonometry  Operator=atan2
  Constant : Constant  Value=pi
  Sum : Sum  Inputs=+-+
  Unwrap : dspsigops/Unwrap  tol=pi  InputProcessing=Columns as channels (frame based)  running=off
  gamma : Outport
  wires:
  e_x/1 -> Atan2/2
  e_y/1 -> Atan2/1
  theta/1 -> Sum/2
  Sum/1 -> gamma/1
  Atan2/1 -> Unwrap/1
  Constant/1 -> Sum/3
  Unwrap/1 -> Sum/1

== system Switching_07/Unicycle 3/Posture Regulation Controller/Subsystem2 ==
  gamma : Inport
  e_theta : Inport  Port=2
  Sum : Sum
  delta : Outport
  wires:
  e_theta/1 -> Sum/2
  Sum/1 -> delta/1
  gamma/1 -> Sum/1

== matlab function Switching_07/Unicycle 2/Posture Regulation Controller/MATLAB Function ==
  data: rho input; v output; w output; gamma input; delta input; PR_k1 parameter; PR_k2 parameter; PR_k3 parameter; tolerance_posture parameter
function [v,w] = fcn(rho, gamma, delta, PR_k1, PR_k2, PR_k3, tolerance_posture)

if abs(rho)<tolerance_posture
    v=0;
    w=0;
else
    v=PR_k1*rho*cos(gamma);
    w=PR_k2*gamma+PR_k1*(cos(gamma)*sin(gamma))/gamma*(gamma+PR_k3*delta);
end

== matlab function Switching_07/Unicycle 3/Posture Regulation Controller/MATLAB Function ==
  data: rho input; v output; w output; gamma input; delta input; PR_k1 parameter; PR_k2 parameter; PR_k3 parameter; tolerance_posture parameter
function [v,w] = fcn(rho, gamma, delta, PR_k1, PR_k2, PR_k3, tolerance_posture)

if abs(rho)<tolerance_posture
    v=0;
    w=0;
else
    v=PR_k1*rho*cos(gamma);
    w=PR_k2*gamma+PR_k1*(cos(gamma)*sin(gamma))/gamma*(gamma+PR_k3*delta);
end

== matlab function Switching_07/Unicycle 2/Output Feedback with Further Derivatives/Subsystem2/MATLAB Function ==
  data: v input; u input; a output; w output; theta_rad input
function [a, w] = fcn(v, u, theta_rad)

T_inv=[cos(theta_rad)       sin(theta_rad);
       -sin(theta_rad)/v    cos(theta_rad)/v];

in=T_inv*u;

a = in(1);
w= in(2);

== matlab function Switching_07/Unicycle 1/Output Feedback with Further Derivatives/Subsystem2/MATLAB Function ==
  data: v input; u input; a output; w output; theta_rad input
function [a, w] = fcn(v, u, theta_rad)

T_inv=[cos(theta_rad)       sin(theta_rad);
       -sin(theta_rad)/v    cos(theta_rad)/v];

in=T_inv*u;

a = in(1);
w= in(2);

== matlab function Switching_07/Unicycle 2/Output Feedback with Further Derivatives/Subsystem2/MATLAB Function1 ==
  data: u input; u output
function u = fcn(u)

if abs(u)<1e-4
    if u>=0
        u=1e-4;
    else
        u=-1e-4;
    end
else
    u=u;
end

== matlab function Switching_07/Swittching Logic ==
  data: switching output; v1 input; v2 input; v3 input; w1 input; w2 input; w3 input; switching_out input
function switching = fcn(v1, v2, v3, w1, w2, w3, switching_out)
if switching_out==1
    switching=1;
else
    if v1==0 && v2==0 && v3==0 && w1==0 && w2==0 && w3==0
        switching = 1; 
    else
        switching = 0; 
    end
end

== matlab function Switching_07/Unicycle 3/Output Feedback with Further Derivatives/Subsystem2/MATLAB Function ==
  data: v input; u input; a output; w output; theta_rad input
function [a, w] = fcn(v, u, theta_rad)

T_inv=[cos(theta_rad)       sin(theta_rad);
       -sin(theta_rad)/v    cos(theta_rad)/v];

in=T_inv*u;

a = in(1);
w= in(2);

== matlab function Switching_07/Unicycle 3/Output Feedback with Further Derivatives/Subsystem2/MATLAB Function1 ==
  data: u input; u output
function u = fcn(u)

if abs(u)<1e-4
    if u>=0
        u=1e-4;
    else
        u=-1e-4;
    end
else
    u=u;
end

== matlab function Switching_07/Unicycle 1/Output Feedback with Further Derivatives/Subsystem2/MATLAB Function1 ==
  data: u input; u output
function u = fcn(u)

if abs(u)<1e-4
    if u>=0
        u=1e-4;
    else
        u=-1e-4;
    end
else
    u=u;
end

== matlab function Switching_07/Unicycle 1/Posture Regulation Controller/MATLAB Function ==
  data: rho input; v output; w output; gamma input; delta input; PR_k1 parameter; PR_k2 parameter; PR_k3 parameter; tolerance_posture parameter
function [v,w] = fcn(rho, gamma, delta, PR_k1, PR_k2, PR_k3, tolerance_posture)

if abs(rho)<tolerance_posture
    v=0;
    w=0;
else
    v=PR_k1*rho*cos(gamma);
    w=PR_k2*gamma+PR_k1*(cos(gamma)*sin(gamma))/gamma*(gamma+PR_k3*delta);
end
